simulink model "TRMS"  (R2020a)
settings: Solver=VariableStepAuto  StartTime=0.0  StopTime=50  RelTol=1e-3  EnableMultiTasking=on
InitFcn:
  | TRMS_Kashirin_Aleksandr
undefined symbols (not defined in the file): A, AlphaH_init, AlphaV_init, B, C, Cd, D, DiscIntNeverNeededParam, E, F, F_aero_m, F_aero_t, g, Gam, J_mr, J_tr, J_v, K_fsfb, k_h, K_int, k_v, L, l_b, l_m, l_t, OmegaH_init, OmegaV_init, P_motor_m, P_motor_t, Phi, Tm, Ts, Tt, Wm_init, Wt_init
libraries: simulink_extras x6, vrlib x1
Description:
  | %% BSD 3-Clause License
  | % This mdl-script, its subroutines and relayted Simulink models are parts of
  | % the course Electrical Drives BL30A1001
  | %==========================================================================
  | % Created 17.10.2015;
  | % Authors: NU <Nikita.Uzhegov@lut.fi>, PP <Pavel.Ponomarev@lut.fi>
  | %
  | %==========================================================================
  | % Distributed under BSD 3-Clause License
  | %
  | % Copyright (c) 2015, Nikita Uzhegov <Nikita.Uzhegov@lut.fi>, Pavel Ponomarev <Pavel.V.Ponomarev@gmail.com>
  | % All rights reserved.
  | %
  | % Redistribution and use in source and binary forms, with or without modification, are permitted provided that the following conditions are met:
  | %
  | % Redistributions of source code must retain the above copyright notice, this list of conditions and the following disclaimer.
  | % Redistributions in binary form must reproduce the above copyright notice, this list of conditions and the following disclaimer in the documentation and/or other materials provided with the distribution.
  | % Neither the name of the <Lappeenranta University of Technology> nor the names of its contributors may be used to endorse or promote products derived from this software without specific prior written permission.
  | %
  | % THIS SOFTWARE IS PROVIDED BY THE COPYRIGHT HOLDERS AND CONTRIBUTORS "AS IS" AND ANY EXPRESS OR IMPLIED WARRANTIES, INCLUDING, BUT NOT LIMITED TO, THE IMPLIED WARRANTIES OF MERCHANTABILITY AND FITNESS FOR A PARTICULAR PURPOSE ARE DISCLAIMED. IN NO EVENT SHALL THE COPYRIGHT HOLDER OR CONTRIBUTORS BE LIABLE FOR ANY DIRECT, INDIRECT, INCIDENTAL, SPECIAL, EXEMPLARY, OR CONSEQUENTIAL DAMAGES (INCLUDING, BUT NOT LIMITED TO, PROCUREMENT OF SUBSTITUTE GOODS OR SERVICES; LOSS OF USE, DATA, OR PROFITS; OR BUSINESS INTERRUPTION) HOWEVER CAUSED AND ON ANY THEORY OF LIABILITY, WHETHER IN CONTRACT, STRICT LIABILITY, OR TORT (INCLUDING NEGLIGENCE OR OTHERWISE) ARISING IN ANY WAY OUT OF THE USE OF THIS SOFTWARE, EVEN IF ADVISED OF THE POSSIBILITY OF SUCH DAMAGE.
settings Model: EnablePacing=on  PacingRate=3  Creator=c0347966  LastModifiedBy=User
settings SolverCC: ZeroCrossControl=DisableAll
settings DataIOCC: LimitDataPoints=on  SaveFormat=Array  SignalLoggingSaveFormat=ModelDataLogs  ReturnWorkspaceOutputs=off
settings OptimizationCC: ExpressionDepthLimit=2147483647  LifeSpan=inf
settings DebuggingCC: UnderspecifiedInitializationDetection=Classic  MergeDetectMultiDrivingBlocksExec=none  SolverPrmCheckMsg=warning  StateNameClashWarn=warning  SFUnexpectedBacktrackingDiag=warning  SFNoUnconditionalDefaultTransitionDiag=warning  SFExecutionAtInitializationDiag=none  ArithmeticOperatorsInVariantConditions=warning
settings HardwareCC: ProdBitPerPointer=32  ProdBitPerSizeT=32  ProdBitPerPtrDiffT=32  ProdLargestAtomicFloat=None  ProdIntDivRoundTo=Undefined  ProdEndianess=Unspecified  ProdWordSize=32  ProdHWDeviceType=32-bit Generic
settings ModelReferenceCC: PropagateSignalLabelsOutOfModel=off
settings SFSimCC: SimUseLocalCustomCode=off  CustomCodeUndefinedFunction=UseInterfaceOnly
settings RTWCC: RTWUseLocalCustomCode=off
settings CodeAppCC: StateflowObjectComments=on
settings GRTTargetCC: TargetLangStandard=C89/C90 (ANSI)  CombineOutputUpdateFcns=off  GRTInterface=on
settings ConfigComp: CovMetricSettings=dw  CovHtmlReporting=on  CovSaveCumulativeToWorkspaceVar=on  CovSaveSingleToWorkspaceVar=on  CovExternalEMLEnable=off  CovSFcnEnable=off
settings SimscapeCC: SimscapeNormalizeSystem=off
settings ConfigurationSet: Description=SimMechanics 2G

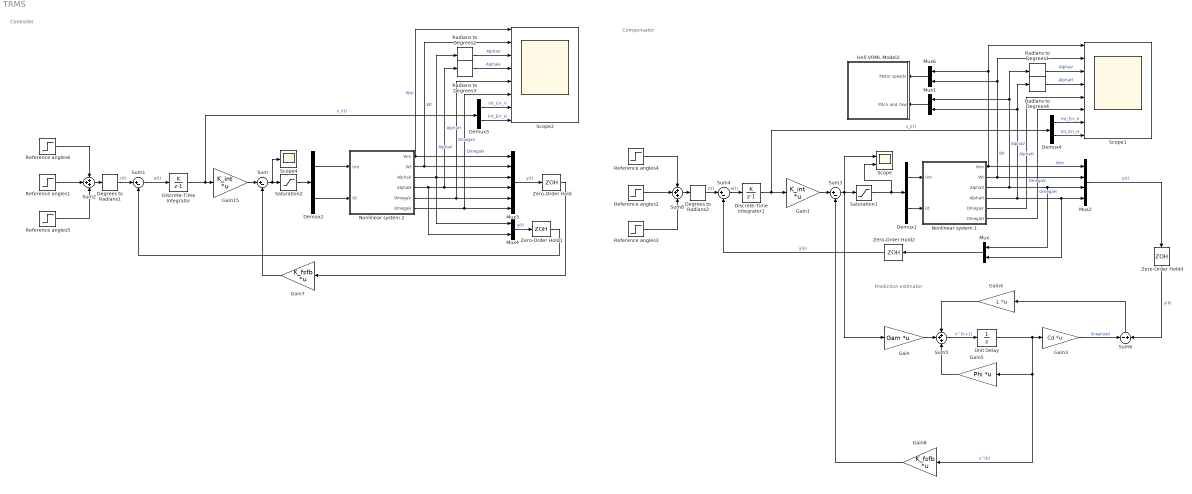
== system TRMS ==
  note: Compensator
  note: Controller
  note: Prediction estimator
  Degrees to Radians1 : simulink_extras/Transformations/Degrees to Radians
  Degrees to Radians2 : simulink_extras/Transformations/Degrees to Radians
  Demux{1..4} (4 alike) : Demux  Outputs=2
  Discrete-Time Integrator : DiscreteIntegrator  IntegratorMethod=Accumulation: Forward Euler  SampleTime=Ts  ICPrevOutput=DiscIntNeverNeededParam  ICPrevScaledInput=DiscIntNeverNeededParam
  Discrete-Time Integrator1 : DiscreteIntegrator  IntegratorMethod=Accumulation: Forward Euler  SampleTime=Ts  ICPrevOutput=DiscIntNeverNeededParam  ICPrevScaledInput=DiscIntNeverNeededParam
  Gain : Gain  Gain=Gam  Multiplication=Matrix(K*u) (u vector)
  Gain1 : Gain  Gain=K_int  Multiplication=Matrix(K*u) (u vector)
  Gain15 : Gain  Gain=K_int  Multiplication=Matrix(K*u) (u vector)
  Gain3 : Gain  Gain=Cd  Multiplication=Matrix(K*u) (u vector)
  Gain4 : Gain  Gain=L  Multiplication=Matrix(K*u) (u vector)
  Gain5 : Gain  Gain=Phi  Multiplication=Matrix(K*u) (u vector)
  Gain7 : Gain  Gain=K_fsfb  Multiplication=Matrix(K*u) (u vector)
  Gain8 : Gain  Gain=K_fsfb  Multiplication=Matrix(K*u) (u vector)
  Heli VRML Model2 : Subsystem
  Mux{,1,4,6} (4 alike) : Mux  Inputs=2
  Mux2 : Mux
  Mux3 : Mux  Inputs=6
  Nonlinear system 1 : Subsystem
  Nonlinear system 2 : Subsystem
  Radians to Degrees{1..4} (4 alike) : simulink_extras/Transformations/Radians to Degrees
  Reference angles1 : Step  Time=0  After=[-5 50]
  Reference angles2 : Step  Time=0  After=[-5 50]
  Reference angles3 : Step  Time=12  After=[-20 -30]  SampleTime=Ts
  Reference angles4 : Step  Time=25  After=[+20 +30]
  Reference angles5 : Step  Time=12  After=[-20 -30]  SampleTime=Ts
  Reference angles6 : Step  Time=25  After=[+20 +30]
  Saturation1 : Saturate  UpperLimit=18  LowerLimit=-18
  Saturation2 : Saturate  UpperLimit=19  LowerLimit=-18
  Scope : Scope  NumInputPorts=2
  Scope1 : Scope  NumInputPorts=8
  Scope2 : Scope  NumInputPorts=8
  Scope4 : Scope
  Sum{,1,3..4} (4 alike) : Sum  Inputs=|+-
  Sum2 : Sum  Inputs=+++
  Sum5 : Sum  Inputs=+++
  Sum6 : Sum  Inputs=-+
  Sum8 : Sum  Inputs=+++
  Unit Delay : UnitDelay  SampleTime=-1  HasFrameUpgradeWarning=on
  Zero-Order Hold{,1..2,4} (4 alike) : ZeroOrderHold  SampleTime=-1
  wires:
  Demux3/2 -> Scope2/8  "Int_Err_H"
  Mux4/1 -> Zero-Order Hold1/1  "y(t)"
  Gain15/1 -> Sum/1
  Nonlinear system 2/5(OmegaV) -> Mux3/5, Scope2/5  "OmegaV"
  Zero-Order Hold1/1 -> Sum1/2
  Saturation2/1 -> Demux2/1
  Nonlinear system 2/1(Wm) -> Scope2/1, Mux3/1  "Wm"
  Nonlinear system 2/3(AlphaV) -> Mux3/3, Mux4/1, Radians to Degrees2/1  "AlphaV"
  Nonlinear system 2/4(AlphaH) -> Mux3/4, Radians to Degrees3/1, Mux4/2  "AlphaH"
  Demux2/2 -> Nonlinear system 2/2(Ut)
  Demux2/1 -> Nonlinear system 2/1(Um)
  Gain7/1 -> Sum/2
  Demux3/1 -> Scope2/7  "Int_Err_V"
  Sum/1 -> Saturation2/1, Scope4/1
  Discrete-Time Integrator/1 -> Demux3/1, Gain15/1  "x_i(t)"
  Nonlinear system 2/2(Wt) -> Scope2/2, Mux3/2  "Wt"
  Mux3/1 -> Zero-Order Hold/1  "y(t)"
  Zero-Order Hold/1 -> Gain7/1
  Nonlinear system 2/6(OmegaH) -> Scope2/6, Mux3/6  "OmegaH"
  Sum1/1 -> Discrete-Time Integrator/1  "e(t)"
  Radians to Degrees2/1 -> Scope2/3  "AlphaV"
  Radians to Degrees3/1 -> Scope2/4  "AlphaH"
  Reference angles2/1 -> Sum8/2
  Mux6/1 -> Heli VRML Model2/1(Motor speeds)
  Demux1/2 -> Nonlinear system 1/2(Ut)
  Sum5/1 -> Unit Delay/1  "x^(k+1)"
  Sum3/1 -> Gain/1, Saturation1/1, Scope/1
  Mux1/1 -> Heli VRML Model2/2(Pitch and Yaw)
  Unit Delay/1 -> Gain8/1, Gain5/1, Gain3/1  "x^(k)"
  Saturation1/1 -> Scope/2, Demux1/1
  Zero-Order Hold4/1 -> Sum6/2  "y(k)"
  Gain4/1 -> Sum5/1
  Gain/1 -> Sum5/2
  Sum4/1 -> Discrete-Time Integrator1/1  "e(t)"
  Gain1/1 -> Sum3/1
  Gain5/1 -> Sum5/3
  Demux4/2 -> Scope1/8  "Int_Err_H"
  Demux1/1 -> Nonlinear system 1/1(Um)
  Discrete-Time Integrator1/1 -> Gain1/1, Demux4/1  "x_i(t)"
  Nonlinear system 1/6(OmegaH) -> Scope1/6  "OmegaH"
  Demux4/1 -> Scope1/7  "Int_Err_V"
  Sum6/1 -> Gain4/1
  Nonlinear system 1/4(AlphaH) -> Mux1/2, Radians to Degrees4/1, Mux/2, Mux2/4  "AlphaH"
  Nonlinear system 1/3(AlphaV) -> Mux/1, Mux2/3, Mux1/1, Radians to Degrees1/1  "AlphaV"
  Gain8/1 -> Sum3/2
  Nonlinear system 1/5(OmegaV) -> Scope1/5  "OmegaV"
  Nonlinear system 1/1(Wm) -> Mux6/1, Scope1/1, Mux2/1  "Wm"
  Mux/1 -> Zero-Order Hold2/1
  Mux2/1 -> Zero-Order Hold4/1  "y(t)"
  Nonlinear system 1/2(Wt) -> Mux6/2, Scope1/2, Mux2/2  "Wt"
  Gain3/1 -> Sum6/1  "linearized"
  Radians to Degrees1/1 -> Scope1/3  "AlphaV"
  Radians to Degrees4/1 -> Scope1/4  "AlphaH"
  Reference angles3/1 -> Sum8/3
  Zero-Order Hold2/1 -> Sum4/2  "y(k)"
  Sum8/1 -> Degrees to Radians2/1
  Degrees to Radians2/1 -> Sum4/1  "r(t)"
  Reference angles4/1 -> Sum8/1
  Reference angles6/1 -> Sum2/1
  Reference angles5/1 -> Sum2/3
  Sum2/1 -> Degrees to Radians1/1
  Reference angles1/1 -> Sum2/2
  Degrees to Radians1/1 -> Sum1/1  "r(t)"

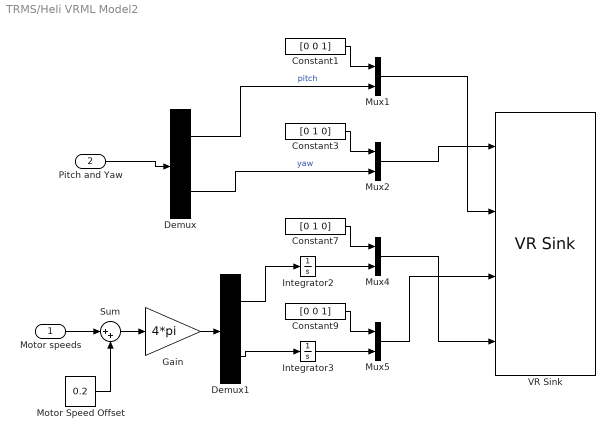
== system TRMS/Heli VRML Model2 ==
  Motor speeds : Inport
  Pitch and Yaw : Inport  Port=2
  Constant1 : Constant  Value=[0 0 1]
  Constant3 : Constant  Value=[0 1 0]
  Constant7 : Constant  Value=[0 1 0]
  Constant9 : Constant  Value=[0 0 1]
  Demux : Demux  Outputs=2
  Demux1 : Demux  Outputs=2
  Gain : Gain  Gain=4*pi
  Integrator2 : Integrator
  Integrator3 : Integrator
  Motor Speed Offset : Constant  Value=0.2
  Mux{1..2,4..5} (4 alike) : Mux  Inputs=2
  Sum : Sum  Inputs=|++
  VR Sink : vrlib/VR Sink  InstantiateOnLoad=on  SampleTime=0.1  ViewEnable=on  RemoteChange=off  RemoteView=off  FieldsWritten=YAW.rotation.4.1.1.double#PITCH.rotation.4.1.1.double#TAILPROP.rotation.4.1.1.double#MAINPROP.rotation.4.1.1.double  WorldFileName=twinrotor.wrl  AutoView=on  VideoDimensions=[]  AllowVariableSize=off
  wires:
  Constant1/1 -> Mux1/1
  Constant3/1 -> Mux2/1
  Constant7/1 -> Mux4/1
  Constant9/1 -> Mux5/1
  Integrator2/1 -> Mux4/2
  Integrator3/1 -> Mux5/2
  Demux/1 -> Mux1/2  "pitch"
  Demux1/1 -> Integrator2/1
  Demux1/2 -> Integrator3/1
  Pitch and Yaw/1 -> Demux/1
  Demux/2 -> Mux2/2  "yaw"
  Gain/1 -> Demux1/1
  Sum/1 -> Gain/1
  Motor speeds/1 -> Sum/1
  Motor Speed Offset/1 -> Sum/2
  Mux4/1 -> VR Sink/4
  Mux5/1 -> VR Sink/3
  Mux2/1 -> VR Sink/1
  Mux1/1 -> VR Sink/2

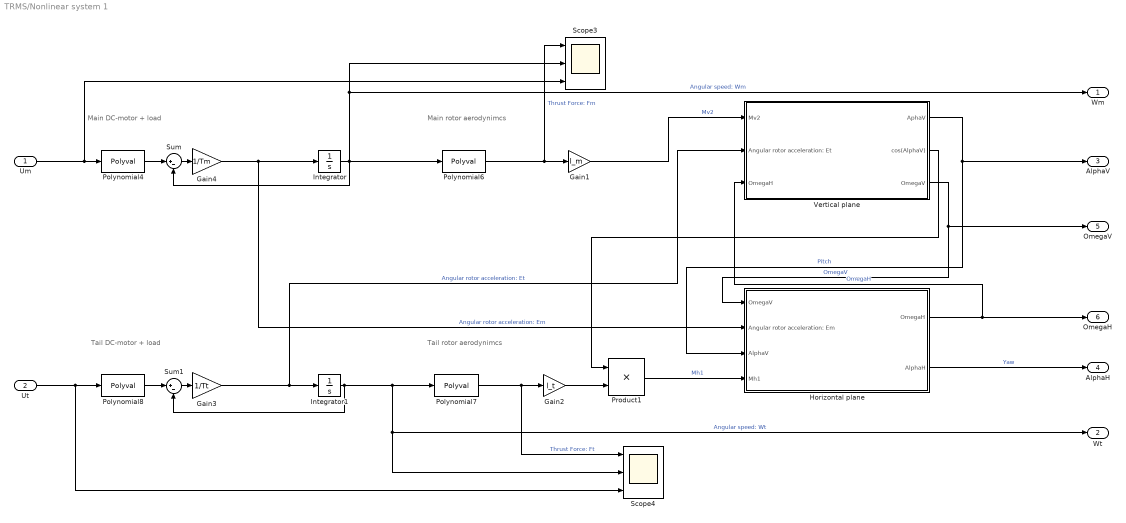
== system TRMS/Nonlinear system 1 ==
  note: Tail rotor aerodynimcs
  note: Main rotor aerodynimcs
  note: Main DC-motor + load
  note: Tail DC-motor + load
  Um : Inport
  Ut : Inport  Port=2
  Gain1 : Gain  Gain=l_m
  Gain2 : Gain  Gain=l_t
  Gain3 : Gain  Gain=1/Tt
  Gain4 : Gain  Gain=1/Tm
  Horizontal plane : Subsystem
  Integrator : Integrator  InitialCondition=Wm_init
  Integrator1 : Integrator  InitialCondition=Wt_init
  Polynomial4 : Polyval  Coefs=P_motor_m
  Polynomial6 : Polyval  Coefs=F_aero_m
  Polynomial7 : Polyval  Coefs=F_aero_t
  Polynomial8 : Polyval  Coefs=P_motor_t
  Product1 : Product
  Scope3 : Scope  NumInputPorts=3
  Scope4 : Scope  NumInputPorts=3
  Sum : Sum  Inputs=|+-
  Sum1 : Sum  Inputs=|+-
  Vertical plane : Subsystem
  Wm : Outport
  Wt : Outport  Port=2
  AlphaV : Outport  Port=3
  AlphaH : Outport  Port=4
  OmegaV : Outport  Port=5
  OmegaH : Outport  Port=6
  wires:
  Gain4/1 -> Horizontal plane/2(Angular rotor acceleration: Em), Integrator/1  "Angular rotor acceleration: Em"
  Gain1/1 -> Vertical plane/1(Mv2)  "Mv2"
  Um/1 -> Polynomial4/1, Scope3/3
  Gain2/1 -> Product1/2
  Integrator1/1 -> Sum1/2, Polynomial7/1, Scope4/2, Wt/1  "Angular speed: Wt"
  Sum1/1 -> Gain3/1
  Polynomial7/1 -> Gain2/1, Scope4/1  "Thrust Force: Ft"
  Polynomial4/1 -> Sum/1
  Horizontal plane/1(OmegaH) -> OmegaH/1, Vertical plane/3(OmegaH)  "OmegaH"
  Sum/1 -> Gain4/1
  Gain3/1 -> Vertical plane/2(Angular rotor acceleration: Et), Integrator1/1  "Angular rotor acceleration: Et"
  Polynomial8/1 -> Sum1/1
  Polynomial6/1 -> Gain1/1, Scope3/1  "Thrust Force: Fm"
  Vertical plane/2(cos(AlphaV)) -> Product1/1
  Integrator/1 -> Wm/1, Scope3/2, Sum/2, Polynomial6/1  "Angular speed: Wm"
  Ut/1 -> Polynomial8/1, Scope4/3
  Vertical plane/3(OmegaV) -> OmegaV/1, Horizontal plane/1(OmegaV)  "OmegaV"
  Product1/1 -> Horizontal plane/4(Mh1)  "Mh1"
  Horizontal plane/2(AlphaH) -> AlphaH/1  "Yaw"
  Vertical plane/1(AphaV) -> AlphaV/1, Horizontal plane/3(AlphaV)  "Pitch"

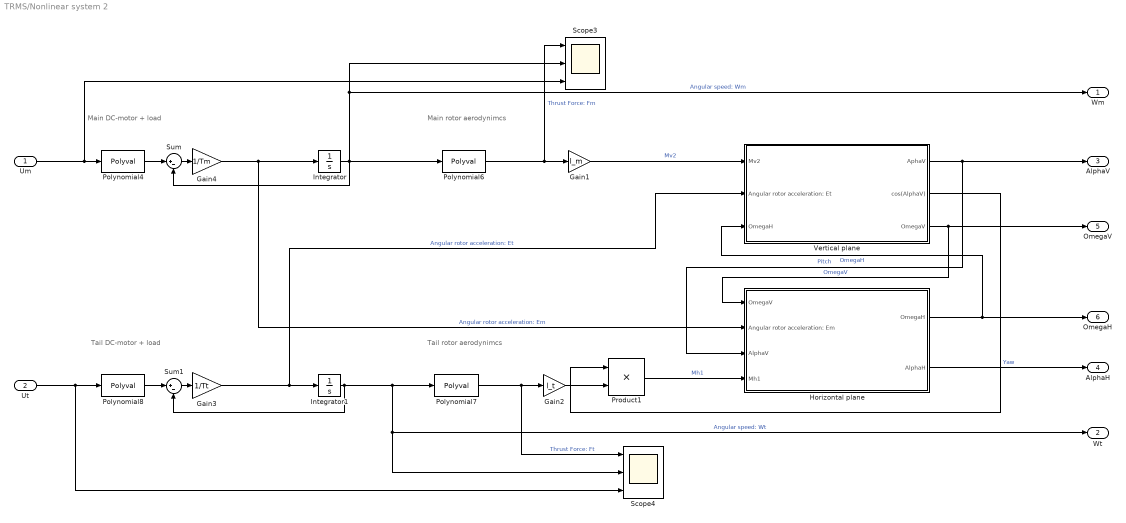
== system TRMS/Nonlinear system 2 ==
  note: Tail rotor aerodynimcs
  note: Main rotor aerodynimcs
  note: Main DC-motor + load
  note: Tail DC-motor + load
  Um : Inport
  Ut : Inport  Port=2
  Gain1 : Gain  Gain=l_m
  Gain2 : Gain  Gain=l_t
  Gain3 : Gain  Gain=1/Tt
  Gain4 : Gain  Gain=1/Tm
  Horizontal plane : Subsystem
  Integrator : Integrator  InitialCondition=Wm_init
  Integrator1 : Integrator  InitialCondition=Wt_init
  Polynomial4 : Polyval  Coefs=P_motor_m
  Polynomial6 : Polyval  Coefs=F_aero_m
  Polynomial7 : Polyval  Coefs=F_aero_t
  Polynomial8 : Polyval  Coefs=P_motor_t
  Product1 : Product
  Scope3 : Scope  NumInputPorts=3
  Scope4 : Scope  NumInputPorts=3
  Sum : Sum  Inputs=|+-
  Sum1 : Sum  Inputs=|+-
  Vertical plane : Subsystem
  Wm : Outport
  Wt : Outport  Port=2
  AlphaV : Outport  Port=3
  AlphaH : Outport  Port=4
  OmegaV : Outport  Port=5
  OmegaH : Outport  Port=6
  wires:
  Gain4/1 -> Horizontal plane/2(Angular rotor acceleration: Em), Integrator/1  "Angular rotor acceleration: Em"
  Gain1/1 -> Vertical plane/1(Mv2)  "Mv2"
  Um/1 -> Polynomial4/1, Scope3/3
  Gain2/1 -> Product1/2
  Integrator1/1 -> Sum1/2, Polynomial7/1, Scope4/2, Wt/1  "Angular speed: Wt"
  Sum1/1 -> Gain3/1
  Polynomial7/1 -> Gain2/1, Scope4/1  "Thrust Force: Ft"
  Polynomial4/1 -> Sum/1
  Horizontal plane/1(OmegaH) -> OmegaH/1, Vertical plane/3(OmegaH)  "OmegaH"
  Sum/1 -> Gain4/1
  Gain3/1 -> Vertical plane/2(Angular rotor acceleration: Et), Integrator1/1  "Angular rotor acceleration: Et"
  Polynomial8/1 -> Sum1/1
  Polynomial6/1 -> Gain1/1, Scope3/1  "Thrust Force: Fm"
  Vertical plane/2(cos(AlphaV)) -> Product1/1
  Integrator/1 -> Wm/1, Scope3/2, Sum/2, Polynomial6/1  "Angular speed: Wm"
  Ut/1 -> Polynomial8/1, Scope4/3
  Vertical plane/3(OmegaV) -> OmegaV/1, Horizontal plane/1(OmegaV)  "OmegaV"
  Product1/1 -> Horizontal plane/4(Mh1)  "Mh1"
  Horizontal plane/2(AlphaH) -> AlphaH/1  "Yaw"
  Vertical plane/1(AphaV) -> AlphaV/1, Horizontal plane/3(AlphaV)  "Pitch"

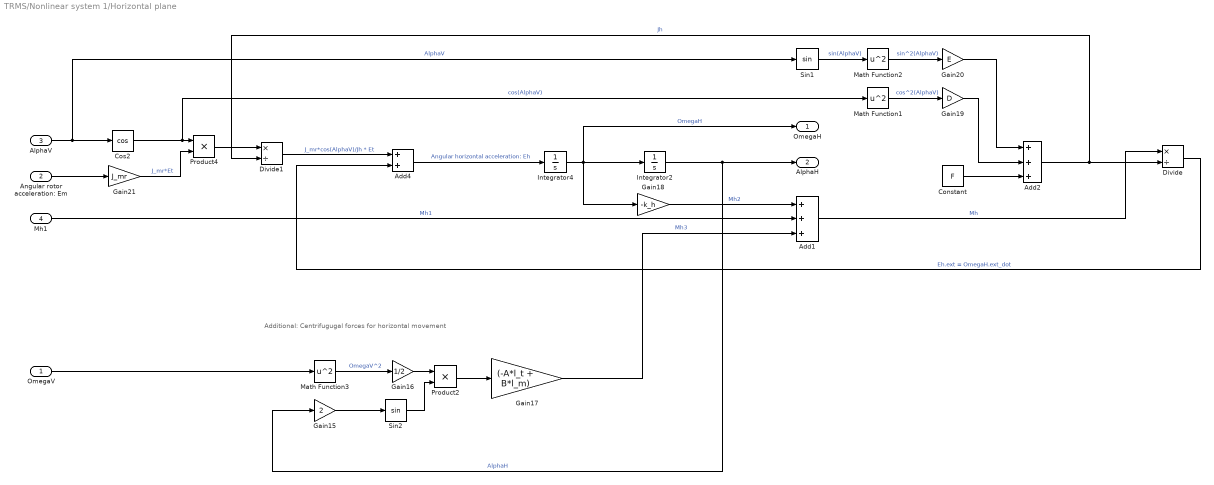
== system TRMS/Nonlinear system 1/Horizontal plane ==
  note: Additional: Centrifugugal forces for horizontal movement
  OmegaV : Inport
  Angular rotor acceleration: Em : Inport  Port=2
  AlphaV : Inport  Port=3
  Mh1 : Inport  Port=4
  Add1 : Sum  Inputs=+++
  Add2 : Sum  Inputs=+++
  Add4 : Sum
  Constant : Constant  Value=F
  Cos2 : Trigonometry  Operator=cos
  Divide : Product  Inputs=*/
  Divide1 : Product  Inputs=*/
  Gain15 : Gain  Gain=2
  Gain16 : Gain  Gain=1/2
  Gain17 : Gain  Gain=(-A*l_t + B*l_m)
  Gain18 : Gain  Gain=-k_h
  Gain19 : Gain  Gain=D
  Gain20 : Gain  Gain=E
  Gain21 : Gain  Gain=J_mr
  Integrator2 : Integrator  InitialCondition=AlphaH_init
  Integrator4 : Integrator  InitialCondition=OmegaH_init
  Math Function1 : Math  Operator=square  SaturateOnIntegerOverflow=on
  Math Function2 : Math  Operator=square  SaturateOnIntegerOverflow=on
  Math Function3 : Math  Operator=square  SaturateOnIntegerOverflow=on
  Product2 : Product
  Product4 : Product
  Sin1 : Trigonometry
  Sin2 : Trigonometry
  OmegaH : Outport
  AlphaH : Outport  Port=2
  wires:
  Add2/1 -> Divide/2, Divide1/2  "Jh"
  Sin2/1 -> Product2/2
  Gain16/1 -> Product2/1
  Angular rotor acceleration: Em/1 -> Gain21/1
  Integrator2/1 -> AlphaH/1, Gain15/1  "AlphaH"
  Sin1/1 -> Math Function2/1  "sin(AlphaV)"
  Divide/1 -> Add4/2  "Eh.ext = OmegaH.ext_dot"
  Constant/1 -> Add2/3
  Integrator4/1 -> OmegaH/1, Gain18/1, Integrator2/1  "OmegaH"
  Math Function1/1 -> Gain19/1  "cos^2(AlphaV)"
  Product4/1 -> Divide1/1
  Divide1/1 -> Add4/1  "J_mr*cos(AlphaV)/Jh * Et"
  OmegaV/1 -> Math Function3/1
  Gain20/1 -> Add2/1
  Math Function2/1 -> Gain20/1  "sin^2(AlphaV)"
  Add1/1 -> Divide/1  "Mh"
  Gain19/1 -> Add2/2
  Mh1/1 -> Add1/2  "Mh1"
  Product2/1 -> Gain17/1
  Gain21/1 -> Product4/2  "J_mr*Et"
  Gain18/1 -> Add1/1  "Mh2"
  Gain15/1 -> Sin2/1
  Math Function3/1 -> Gain16/1  "OmegaV^2"
  Add4/1 -> Integrator4/1  "Angular horizontal acceleration: Eh"
  Cos2/1 -> Math Function1/1, Product4/1  "cos(AlphaV)"
  AlphaV/1 -> Sin1/1, Cos2/1  "AlphaV"
  Gain17/1 -> Add1/3  "Mh3"

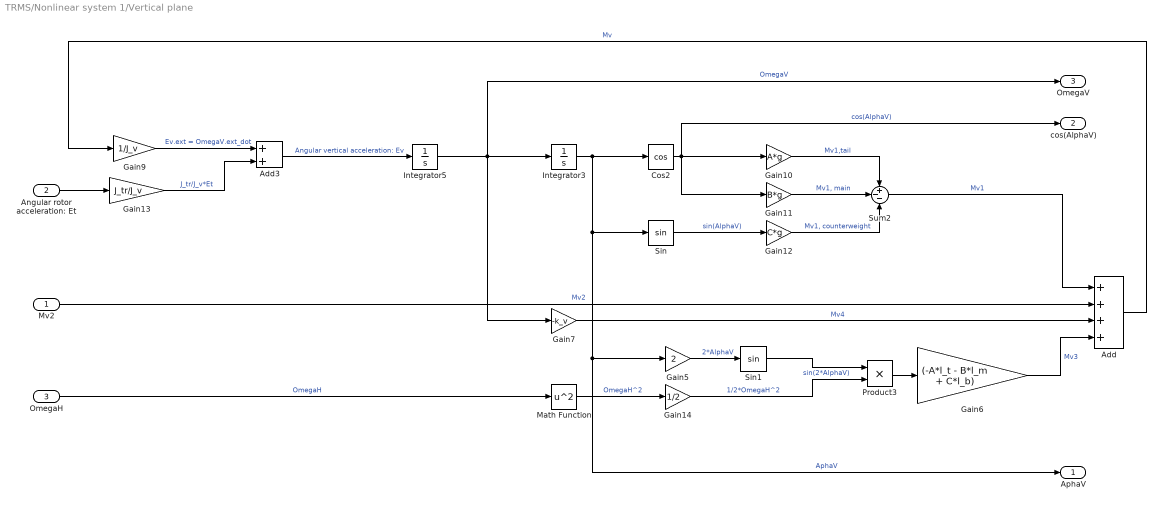
== system TRMS/Nonlinear system 1/Vertical plane ==
  Mv2 : Inport
  Angular rotor acceleration: Et : Inport  Port=2
  OmegaH : Inport  Port=3
  Add : Sum  Inputs=++++
  Add3 : Sum
  Cos2 : Trigonometry  Operator=cos
  Gain10 : Gain  Gain=A*g
  Gain11 : Gain  Gain=B*g
  Gain12 : Gain  Gain=C*g
  Gain13 : Gain  Gain=J_tr/J_v
  Gain14 : Gain  Gain=1/2
  Gain5 : Gain  Gain=2
  Gain6 : Gain  Gain=(-A*l_t - B*l_m + C*l_b)
  Gain7 : Gain  Gain=-k_v
  Gain9 : Gain  Gain=1/J_v
  Integrator3 : Integrator  InitialCondition=AlphaV_init
  Integrator5 : Integrator  InitialCondition=OmegaV_init
  Math Function : Math  Operator=square  SaturateOnIntegerOverflow=on
  Product3 : Product
  Sin : Trigonometry
  Sin1 : Trigonometry
  Sum2 : Sum  Inputs=+--
  AphaV : Outport
  cos(AlphaV) : Outport  Port=2
  OmegaV : Outport  Port=3
  wires:
  OmegaH/1 -> Math Function/1  "OmegaH"
  Integrator5/1 -> OmegaV/1, Gain7/1, Integrator3/1  "OmegaV"
  Cos2/1 -> Gain11/1, cos(AlphaV)/1, Gain10/1  "cos(AlphaV)"
  Gain9/1 -> Add3/1  "Ev.ext = OmegaV.ext_dot"
  Math Function/1 -> Gain14/1  "OmegaH^2"
  Add/1 -> Gain9/1  "Mv"
  Gain5/1 -> Sin1/1  "2*AlphaV"
  Integrator3/1 -> Cos2/1, Sin/1, Gain5/1, AphaV/1  "AphaV"
  Gain13/1 -> Add3/2  "J_tr/J_v*Et"
  Add3/1 -> Integrator5/1  "Angular vertical acceleration: Ev"
  Product3/1 -> Gain6/1
  Gain6/1 -> Add/4  "Mv3"
  Gain11/1 -> Sum2/2  "Mv1, main"
  Gain14/1 -> Product3/2  "1/2*OmegaH^2"
  Gain12/1 -> Sum2/3  "Mv1, counterweight"
  Sin/1 -> Gain12/1  "sin(AlphaV)"
  Sum2/1 -> Add/1  "Mv1"
  Gain10/1 -> Sum2/1  "Mv1,tail"
  Gain7/1 -> Add/3  "Mv4"
  Mv2/1 -> Add/2  "Mv2"
  Angular rotor acceleration: Et/1 -> Gain13/1
  Sin1/1 -> Product3/1  "sin(2*AlphaV)"

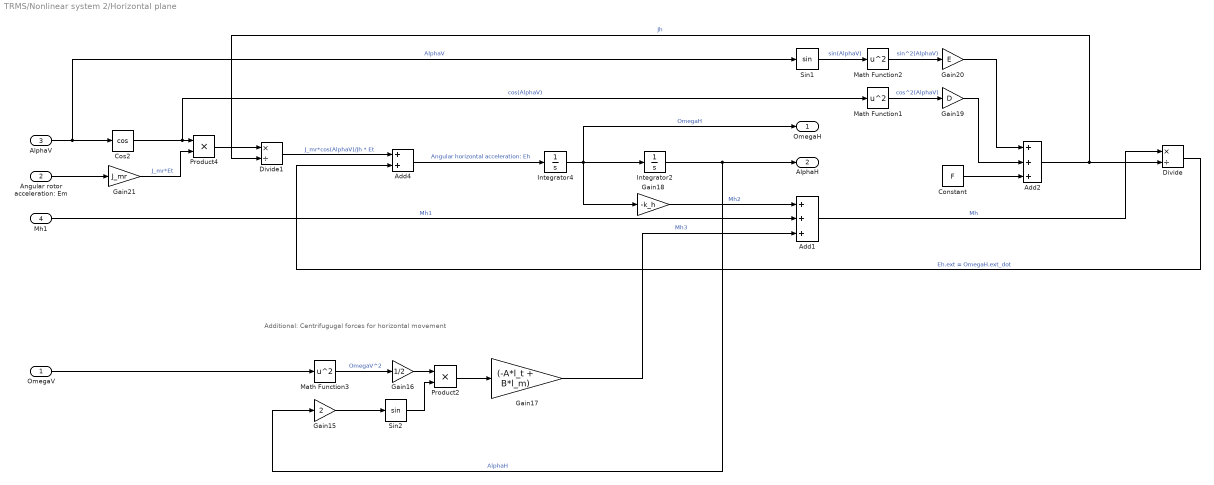
== system TRMS/Nonlinear system 2/Horizontal plane ==
  note: Additional: Centrifugugal forces for horizontal movement
  OmegaV : Inport
  Angular rotor acceleration: Em : Inport  Port=2
  AlphaV : Inport  Port=3
  Mh1 : Inport  Port=4
  Add1 : Sum  Inputs=+++
  Add2 : Sum  Inputs=+++
  Add4 : Sum
  Constant : Constant  Value=F
  Cos2 : Trigonometry  Operator=cos
  Divide : Product  Inputs=*/
  Divide1 : Product  Inputs=*/
  Gain15 : Gain  Gain=2
  Gain16 : Gain  Gain=1/2
  Gain17 : Gain  Gain=(-A*l_t + B*l_m)
  Gain18 : Gain  Gain=-k_h
  Gain19 : Gain  Gain=D
  Gain20 : Gain  Gain=E
  Gain21 : Gain  Gain=J_mr
  Integrator2 : Integrator  InitialCondition=AlphaH_init
  Integrator4 : Integrator  InitialCondition=OmegaH_init
  Math Function1 : Math  Operator=square  SaturateOnIntegerOverflow=on
  Math Function2 : Math  Operator=square  SaturateOnIntegerOverflow=on
  Math Function3 : Math  Operator=square  SaturateOnIntegerOverflow=on
  Product2 : Product
  Product4 : Product
  Sin1 : Trigonometry
  Sin2 : Trigonometry
  OmegaH : Outport
  AlphaH : Outport  Port=2
  wires:
  Add2/1 -> Divide/2, Divide1/2  "Jh"
  Sin2/1 -> Product2/2
  Gain16/1 -> Product2/1
  Angular rotor acceleration: Em/1 -> Gain21/1
  Integrator2/1 -> AlphaH/1, Gain15/1  "AlphaH"
  Sin1/1 -> Math Function2/1  "sin(AlphaV)"
  Divide/1 -> Add4/2  "Eh.ext = OmegaH.ext_dot"
  Constant/1 -> Add2/3
  Integrator4/1 -> OmegaH/1, Gain18/1, Integrator2/1  "OmegaH"
  Math Function1/1 -> Gain19/1  "cos^2(AlphaV)"
  Product4/1 -> Divide1/1
  Divide1/1 -> Add4/1  "J_mr*cos(AlphaV)/Jh * Et"
  OmegaV/1 -> Math Function3/1
  Gain20/1 -> Add2/1
  Math Function2/1 -> Gain20/1  "sin^2(AlphaV)"
  Add1/1 -> Divide/1  "Mh"
  Gain19/1 -> Add2/2
  Mh1/1 -> Add1/2  "Mh1"
  Product2/1 -> Gain17/1
  Gain21/1 -> Product4/2  "J_mr*Et"
  Gain18/1 -> Add1/1  "Mh2"
  Gain15/1 -> Sin2/1
  Math Function3/1 -> Gain16/1  "OmegaV^2"
  Add4/1 -> Integrator4/1  "Angular horizontal acceleration: Eh"
  Cos2/1 -> Math Function1/1, Product4/1  "cos(AlphaV)"
  AlphaV/1 -> Sin1/1, Cos2/1  "AlphaV"
  Gain17/1 -> Add1/3  "Mh3"

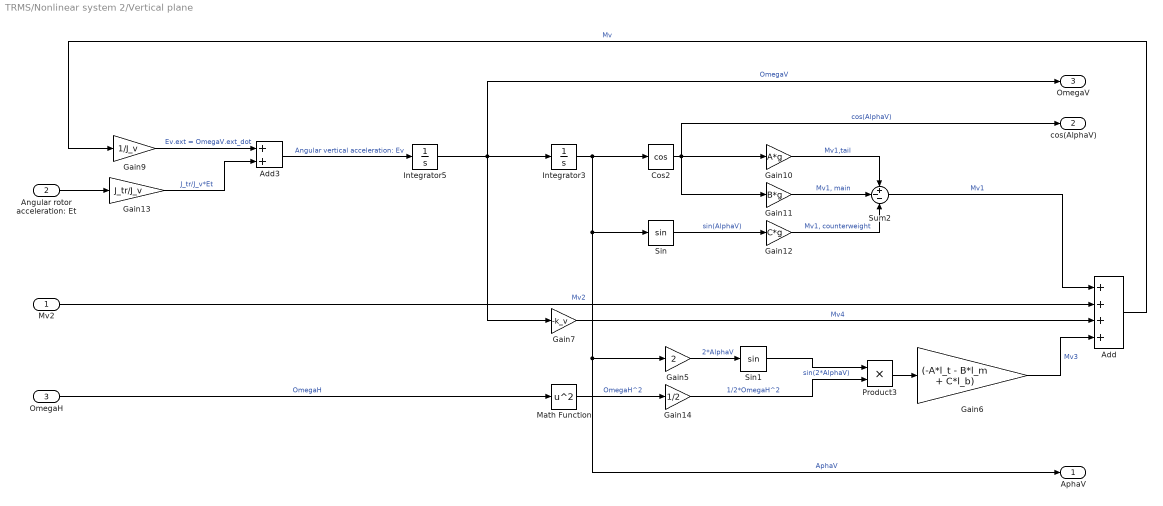
== system TRMS/Nonlinear system 2/Vertical plane ==
  Mv2 : Inport
  Angular rotor acceleration: Et : Inport  Port=2
  OmegaH : Inport  Port=3
  Add : Sum  Inputs=++++
  Add3 : Sum
  Cos2 : Trigonometry  Operator=cos
  Gain10 : Gain  Gain=A*g
  Gain11 : Gain  Gain=B*g
  Gain12 : Gain  Gain=C*g
  Gain13 : Gain  Gain=J_tr/J_v
  Gain14 : Gain  Gain=1/2
  Gain5 : Gain  Gain=2
  Gain6 : Gain  Gain=(-A*l_t - B*l_m + C*l_b)
  Gain7 : Gain  Gain=-k_v
  Gain9 : Gain  Gain=1/J_v
  Integrator3 : Integrator  InitialCondition=AlphaV_init
  Integrator5 : Integrator  InitialCondition=OmegaV_init
  Math Function : Math  Operator=square  SaturateOnIntegerOverflow=on
  Product3 : Product
  Sin : Trigonometry
  Sin1 : Trigonometry
  Sum2 : Sum  Inputs=+--
  AphaV : Outport
  cos(AlphaV) : Outport  Port=2
  OmegaV : Outport  Port=3
  wires:
  OmegaH/1 -> Math Function/1  "OmegaH"
  Integrator5/1 -> OmegaV/1, Gain7/1, Integrator3/1  "OmegaV"
  Cos2/1 -> Gain11/1, cos(AlphaV)/1, Gain10/1  "cos(AlphaV)"
  Gain9/1 -> Add3/1  "Ev.ext = OmegaV.ext_dot"
  Math Function/1 -> Gain14/1  "OmegaH^2"
  Add/1 -> Gain9/1  "Mv"
  Gain5/1 -> Sin1/1  "2*AlphaV"
  Integrator3/1 -> Cos2/1, Sin/1, Gain5/1, AphaV/1  "AphaV"
  Gain13/1 -> Add3/2  "J_tr/J_v*Et"
  Add3/1 -> Integrator5/1  "Angular vertical acceleration: Ev"
  Product3/1 -> Gain6/1
  Gain6/1 -> Add/4  "Mv3"
  Gain11/1 -> Sum2/2  "Mv1, main"
  Gain14/1 -> Product3/2  "1/2*OmegaH^2"
  Gain12/1 -> Sum2/3  "Mv1, counterweight"
  Sin/1 -> Gain12/1  "sin(AlphaV)"
  Sum2/1 -> Add/1  "Mv1"
  Gain10/1 -> Sum2/1  "Mv1,tail"
  Gain7/1 -> Add/3  "Mv4"
  Mv2/1 -> Add/2  "Mv2"
  Angular rotor acceleration: Et/1 -> Gain13/1
  Sin1/1 -> Product3/1  "sin(2*AlphaV)"
